simulink model "sampleModel2034"  (R2023a)
settings: Solver=VariableStepAuto  StartTime=0.0  StopTime=10.0  RelTol=1e-3
libraries: hdlsllib x3, simulink x1
settings Model: Creator=user1  LastModifiedBy=user1

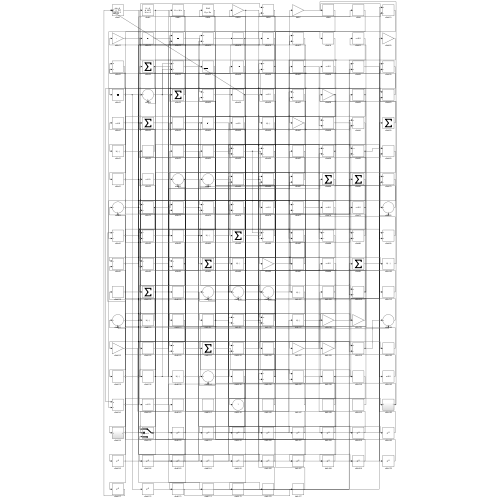
[thumbnail: Simulink's stored preview of the top-level diagram]
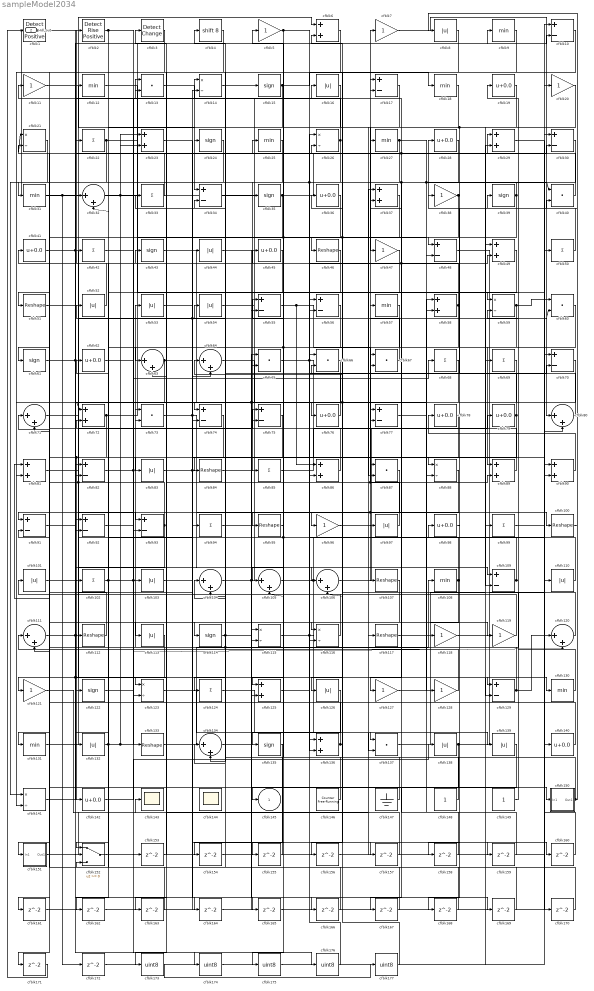
== system sampleModel2034 ==
  cfblk1 : hdlsllib/Logic and Bit Operations/Detect Rise Positive  vinit=0  OutDataTypeStr=uint8
  cfblk{10,17,30,34,48,55..56,70,74..75,77,82,91..93,109,129} (17 alike) : Sum  Inputs=+-  OutDataTypeStr=uint8
  cfblk{46,51,84,95,100,107,112,117,133} (9 alike) : Reshape
  cfblk{8,16,44,52..54,83,97,101,103,110,113,126,132,138..139} (16 alike) : Abs  OutDataTypeStr=uint8  SaturateOnIntegerOverflow=off
  cfblk{22,33,42,50,68..69,85,94,99,102,124} (11 alike) : Sum  Inputs=+  OutDataTypeStr=uint8
  cfblk{32,63..64,71,80,104..106,111,120,134} (11 alike) : Sum  Inputs=|++  OutDataTypeStr=uint8
  cfblk{9,12,18,25,27,31,57,108,130..131} (10 alike) : MinMax  OutDataTypeStr=uint8
  cfblk{5,7,11,20,38,47,96,118..119,121,127..128} (12 alike) : Gain  OutDataTypeStr=uint8
  cfblk{15,24,35,39,43,61,114,122,135} (9 alike) : Signum
  cfblk{14,21,26,59,88,115..116,123,141} (9 alike) : Product  Inputs=*/  OutDataTypeStr=uint8  RndMeth=Zero  SaturateOnIntegerOverflow=on
  cfblk{6,23,29,37,49,58,72,81,86,89..90,125,136} (13 alike) : Sum  OutDataTypeStr=uint8
  cfblk{13,40,60,65..67,73,87,137} (9 alike) : DotProduct  OutDataTypeStr=uint8
  cfblk{19,28,36,41,45,62,76,78..79,98,140,142} (12 alike) : Bias  Bias=0.0  SaturateOnIntegerOverflow=off
  cfblk143 : Scope
  cfblk144 : Scope
      settings: Floating=on
  cfblk146 : hdlsllib/Sources/Counter Free-Running  NumBits=16  tsamp=-1
  cfblk147 : Ground
  cfblk148 : Constant  OutDataTypeStr=uint8  SampleTime=-1
  cfblk149 : Constant  OutDataTypeStr=uint8  SampleTime=-1
  cfblk150 : Subsystem
      settings: LibrarySourceBlock=|
      | hdlsllib/Ports &
      | Subsystems/Subsystem
  cfblk151 : Subsystem
      settings: LibrarySourceBlock=|
      | hdlsllib/Ports &
      | Subsystems/Subsystem
  cfblk152 : Switch  OutDataTypeStr=uint8  SaturateOnIntegerOverflow=off  InputSameDT=off
  cfblk{153..172} (20 alike) : Delay  SampleTime=1
  cfblk{173..177} (5 alike) : DataTypeConversion  OutDataTypeStr=uint8  SaturateOnIntegerOverflow=off  RndMeth=Floor
  cfblk2 : hdlsllib/Logic and Bit Operations/Detect Rise Positive  vinit=0  OutDataTypeStr=uint8
  cfblk3 : simulink/Logic and Bit Operations/Detect Change  vinit=0  OutDataTypeStr=uint8
      settings: LibrarySourceBlock=|
      | hdlsllib/Logic and Bit
      | Operations/Detect
      | Change
  cfblk4 : ArithShift  BitShiftNumber=8
  cfblk145 : Outport  OutDataTypeStr=uint8  VectorParamsAs1DForOutWhenUnconnected=off
  Hdl_out : Outport  Port=2  OutDataTypeStr=uint8
  wires:
  cfblk119/1 -> cfblk101/1
  cfblk115/1 -> cfblk137/1, cfblk70/2
  cfblk72/1 -> cfblk9/1, cfblk131/1
  cfblk93/1 -> cfblk6/1, cfblk71/2, cfblk152/1
  cfblk48/1 -> cfblk114/1
  cfblk146/1 -> cfblk81/1, cfblk52/1
  cfblk129/1 -> cfblk53/1, cfblk120/1
  cfblk128/1 -> cfblk111/1
  cfblk33/1 -> cfblk2/1
  cfblk51/1 -> cfblk109/1
  cfblk78/1 -> cfblk142/1, cfblk82/2
  cfblk28/1 -> cfblk83/1
  cfblk104/1 -> cfblk16/1, cfblk106/1
  cfblk4/1 -> cfblk123/1
  cfblk31/1 -> cfblk172/1, cfblk176/1
  cfblk74/1 -> cfblk113/1
  cfblk82/1 -> cfblk14/1, cfblk120/2
  cfblk97/1 -> cfblk7/1, cfblk13/1
  cfblk52/1 -> cfblk22/1
  cfblk54/1 -> cfblk59/1
  cfblk89/1 -> cfblk41/1
  cfblk65/1 -> cfblk88/1, cfblk49/2
  cfblk41/1 -> cfblk130/1, cfblk30/2
  cfblk133/1 -> cfblk108/1
  cfblk34/1 -> cfblk85/1
  cfblk7/1 -> cfblk80/1
  cfblk10/1 -> cfblk74/1
  cfblk32/1 -> cfblk110/1, cfblk23/1
  cfblk14/1 -> cfblk15/1
  cfblk149/1 -> cfblk59/2
  cfblk118/1 -> cfblk10/1
  cfblk50/1 -> cfblk28/1
  cfblk43/1 -> cfblk76/1
  cfblk123/1 -> cfblk137/2
  cfblk18/1 -> cfblk47/1
  cfblk114/1 -> cfblk4/1, cfblk157/1
  cfblk83/1 -> cfblk116/2, cfblk166/1
  cfblk61/1 -> cfblk129/2, cfblk165/1, cfblk13/2
  cfblk38/1 -> cfblk105/1, cfblk93/1, cfblk168/1
  cfblk120/1 -> cfblk64/1
  cfblk63/1 -> cfblk26/2, cfblk60/2, cfblk81/2
  cfblk150/1(Out1) -> cfblk6/2, cfblk40/2
  cfblk20/1 -> cfblk109/2
  cfblk13/1 -> cfblk34/1
  cfblk81/1 -> cfblk75/1
  cfblk35/1 -> cfblk29/1, cfblk51/1, Hdl_out/1
  cfblk22/1 -> cfblk88/2, cfblk152/2
  cfblk36/1 -> cfblk46/1
  cfblk121/1 -> cfblk143/1
  cfblk56/1 -> cfblk63/1
  cfblk85/1 -> cfblk29/2
  cfblk59/1 -> cfblk89/1, cfblk60/1
  cfblk49/1 -> cfblk135/1
  cfblk102/1 -> cfblk125/2, cfblk67/2, cfblk162/1
  cfblk131/1 -> cfblk54/1
  cfblk5/1 -> cfblk105/2, cfblk100/1
  cfblk147/1 -> cfblk55/1
  cfblk137/1 -> cfblk49/1
  cfblk75/1 -> cfblk92/1
  cfblk88/1 -> cfblk91/1
  cfblk90/1 -> cfblk78/1
  cfblk70/1 -> cfblk126/1, cfblk72/1
  cfblk151/1(Out1) -> cfblk117/1
  cfblk106/1 -> cfblk79/1
  cfblk60/1 -> cfblk122/1
  cfblk138/1 -> cfblk50/1, cfblk167/1
  cfblk19/1 -> cfblk48/1, cfblk87/2
  cfblk109/1 -> cfblk39/1, cfblk67/1
  cfblk55/1 -> cfblk107/1, cfblk86/1
  cfblk29/1 -> cfblk140/1
  cfblk112/1 -> cfblk71/1
  cfblk71/1 -> cfblk123/2
  cfblk96/1 -> cfblk89/2
  cfblk84/1 -> cfblk150/1(In1)
  cfblk101/1 -> cfblk44/1
  cfblk86/1 -> cfblk34/2
  cfblk77/1 -> cfblk58/2
  cfblk105/1 -> cfblk129/1, cfblk30/1
  cfblk117/1 -> cfblk119/1
  cfblk21/1 -> cfblk141/1
  cfblk68/1 -> cfblk75/2, cfblk92/2
  cfblk107/1 -> cfblk124/1
  cfblk100/1 -> cfblk8/1
  cfblk95/1 -> cfblk45/1
  cfblk1/1 -> cfblk77/1
  cfblk12/1 -> cfblk48/2
  cfblk16/1 -> cfblk56/2
  cfblk25/1 -> cfblk102/1
  cfblk40/1 -> cfblk21/1, cfblk17/2
  cfblk67/1 -> cfblk57/1
  cfblk122/1 -> cfblk68/1
  cfblk92/1 -> cfblk133/1
  cfblk47/1 -> cfblk132/1
  cfblk111/1 -> cfblk14/2, cfblk10/2, cfblk164/1
  cfblk37/1 -> cfblk104/2, cfblk106/2
  cfblk64/1 -> cfblk128/1
  cfblk79/1 -> cfblk33/1, cfblk82/1
  cfblk142/1 -> cfblk138/1
  cfblk2/1 -> cfblk32/2, cfblk174/1
  cfblk73/1 -> cfblk136/2, cfblk87/1
  cfblk125/1 -> cfblk98/1
  cfblk6/1 -> cfblk61/1
  cfblk30/1 -> cfblk127/1, cfblk93/2
  cfblk8/1 -> cfblk116/1
  cfblk26/1 -> cfblk134/2, cfblk86/2, cfblk11/1
  cfblk108/1 -> cfblk121/1, cfblk62/1
  cfblk116/1 -> cfblk43/1
  cfblk42/1 -> cfblk103/1
  cfblk15/1 -> cfblk112/1, cfblk18/1
  cfblk134/1 -> cfblk65/1
  cfblk141/1 -> cfblk17/1
  cfblk130/1 -> cfblk19/1
  cfblk24/1 -> cfblk151/1(In1)
  cfblk3/1 -> cfblk141/2
  cfblk23/1 -> cfblk74/2
  cfblk11/1 -> cfblk24/1
  cfblk80/1 -> cfblk38/1
  cfblk127/1 -> cfblk118/1
  cfblk17/1 -> cfblk145/1
  cfblk124/1 -> cfblk139/1
  cfblk45/1 -> cfblk55/2
  cfblk91/1 -> cfblk32/1
  cfblk53/1 -> cfblk94/1
  cfblk58/1 -> cfblk95/1, cfblk84/1, cfblk37/2, cfblk21/2
  cfblk87/1 -> cfblk125/1, cfblk97/1
  cfblk46/1 -> cfblk115/2
  cfblk110/1 -> cfblk73/1, cfblk5/1
  cfblk140/1 -> cfblk111/2
  cfblk148/1 -> cfblk27/1
  cfblk27/1 -> cfblk40/1, cfblk90/2, cfblk35/1
  cfblk76/1 -> cfblk12/1
  cfblk39/1 -> cfblk31/1, cfblk96/1
  cfblk152/1 -> cfblk90/1
  cfblk132/1 -> cfblk23/2, cfblk25/1, cfblk42/1
  cfblk136/1 -> cfblk3/1, cfblk36/1
  cfblk62/1 -> cfblk153/1
  cfblk153/1 -> cfblk63/2
  cfblk135/1 -> cfblk154/1
  cfblk154/1 -> cfblk136/1
  cfblk126/1 -> cfblk155/1
  cfblk155/1 -> cfblk115/1
  cfblk9/1 -> cfblk156/1
  cfblk156/1 -> cfblk37/1
  cfblk157/1 -> cfblk73/2
  cfblk98/1 -> cfblk158/1
  cfblk158/1 -> cfblk58/1
  cfblk94/1 -> cfblk159/1
  cfblk159/1 -> cfblk77/2
  cfblk103/1 -> cfblk160/1
  cfblk160/1 -> cfblk70/1
  cfblk113/1 -> cfblk161/1
  cfblk161/1 -> cfblk26/1
  cfblk162/1 -> cfblk64/2
  cfblk57/1 -> cfblk163/1
  cfblk163/1 -> cfblk91/2
  cfblk164/1 -> cfblk65/2
  cfblk165/1 -> cfblk80/2
  cfblk166/1 -> cfblk134/1
  cfblk167/1 -> cfblk152/3
  cfblk168/1 -> cfblk72/2
  cfblk44/1 -> cfblk169/1
  cfblk169/1 -> cfblk56/1
  cfblk99/1 -> cfblk170/1
  cfblk170/1 -> cfblk104/1
  cfblk139/1 -> cfblk171/1
  cfblk171/1 -> cfblk1/1
  cfblk172/1 -> cfblk20/1
  cfblk69/1 -> cfblk173/1
  cfblk174/1 -> cfblk69/1
  cfblk66/1 -> cfblk175/1
  cfblk175/1 -> cfblk99/1
  cfblk176/1 -> cfblk66/1
  cfblk173/1 -> cfblk177/1
  cfblk177/1 -> cfblk66/2

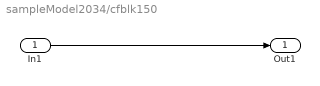
== system sampleModel2034/cfblk150 ==
  In1 : Inport
  Out1 : Outport
  wires:
  In1/1 -> Out1/1

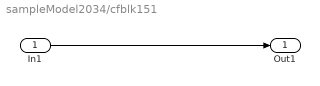
== system sampleModel2034/cfblk151 ==
  In1 : Inport
  Out1 : Outport
  wires:
  In1/1 -> Out1/1
